simulink model "test_multi_bram_Delay"  (Simulink 7.6)
settings: Solver=ode45  StartTime=0.0  StopTime=10.0  RelTol=1e-3
libraries: xbsIndex_r4 x32, monroe_library x2, xps_library x1
settings Model: Creator=monroe  LastModifiedBy=monroe

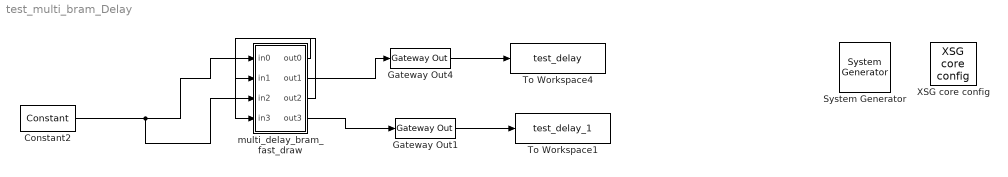
== system test_multi_bram_Delay ==
  " System Generator" : xbsIndex_r4/ System Generator  Tag=genX  SystemSampleTime=-1  xilinxfamily=virtex5  part=xc5vsx95t  speed=-1  package=ff1136  synthesis_tool=XST  clock_wrapper=Clock Enables  directory=./spec_2pol_4kw_6tap_pfb/sysgen  testbench=off  simulink_period=1  sysclk_period=2.6667  dcm_input_clock_period=100  incr_netlist=off  trim_vbits=Everywhere in SubSystem  dbl_ovrd=According to Block Masks  core_generation=According to Block Masks  run_coregen=off  deprecated_control=off  eval_field=0  block_type=sysgen
      settings: block_version=11.4
  Constant2 : xbsIndex_r4/Constant  arith_type=Signed (2's comp)  const=0.9  n_bits=8  bin_pt=7  explicit_period=on  period=1  equ=P=C  opselect=C  inp2=PCIN>>17  opr=+  inp1=P  carry=CIN  dbl_ovrd=off  block_type=constant
  Gateway Out1 : xbsIndex_r4/Gateway Out  hdl_port=on  timing_constraint=None  locs_specified=off  LOCs={}  block_type=gatewayout
      settings: infoedit="Gateway out block.  Converts Xilinx fixed point inputs into ouputs of type Simulink integer, double, or fixed point.<br><br>Hardware notes:  In hardware these blocks become top level output ports or are discarded, depending on how they are configured."  block_version=12.3
  Gateway Out4 : xbsIndex_r4/Gateway Out  hdl_port=on  timing_constraint=None  locs_specified=off  LOCs={}  block_type=gatewayout
      settings: infoedit="Gateway out block.  Converts Xilinx fixed point inputs into ouputs of type Simulink integer, double, or fixed point.<br><br>Hardware notes:  In hardware these blocks become top level output ports or are discarded, depending on how they are configured."  block_version=12.3
  To Workspace1 : ToWorkspace  VariableName=test_delay_1  SampleTime=-1  SaveFormat=Structure
  To Workspace4 : ToWorkspace  VariableName=test_delay  SampleTime=-1  SaveFormat=Structure
  XSG core config : xps_library/XSG core config  Tag=xps:xsg  SystemSampleTime=-1  hw_sys=ROACH:sx95t  ibob_linux=off  clk_src=adc0_clk  iBOB_clk_src=sys_clk  BEE2_ctrl_clk_src=sys_clk  BEE2_usr_clk_src=sys_clk  ROACH_clk_src=adc0_clk  CORR_clk_src=sys_clk  gpio_clk_io_group=iBOB:sma  gpio_clk_bit_index=0  clk_rate=375  sample_period=1  synthesis_tool=XST  mpc_type=powerpc440_ext
  multi_delay_bram_fast_draw : Subsystem
  wires:
  multi_delay_bram_fast_draw/3(out2) -> multi_delay_bram_fast_draw/4(in3)
  multi_delay_bram_fast_draw/1(out0) -> multi_delay_bram_fast_draw/2(in1)
  Constant2/1 -> multi_delay_bram_fast_draw/1(in0), multi_delay_bram_fast_draw/3(in2)
  Gateway Out4/1 -> To Workspace4/1
  Gateway Out1/1 -> To Workspace1/1
  multi_delay_bram_fast_draw/2(out1) -> Gateway Out4/1
  multi_delay_bram_fast_draw/4(out3) -> Gateway Out1/1

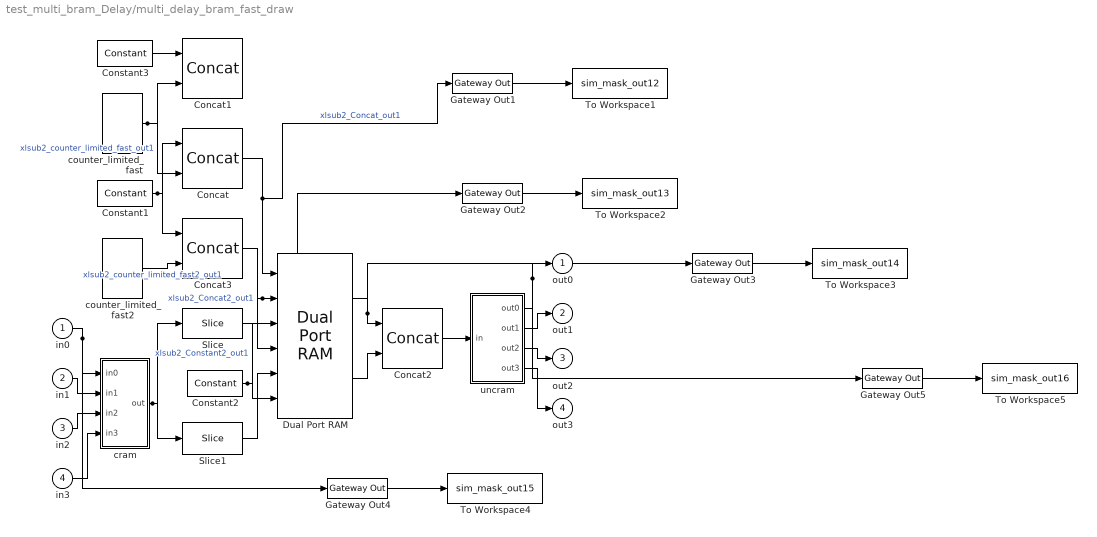
== system test_multi_bram_Delay/multi_delay_bram_fast_draw ==
  in0 : Inport
  in1 : Inport  Port=2
  in2 : Inport  Port=3
  in3 : Inport  Port=4
  Concat{,1..3} (4 alike) : xbsIndex_r4/Concat  num_inputs=2  dbl_ovrd=off  block_type=concat
  Constant1 : xbsIndex_r4/Constant  arith_type=Boolean  const=1  n_bits=1  bin_pt=0  explicit_period=on  period=1  equ=P=C  opselect=C  inp2=PCIN>>17  opr=+  inp1=P  carry=CIN  dbl_ovrd=off  block_type=constant
  Constant2 : xbsIndex_r4/Constant  arith_type=Boolean  const=1  n_bits=1  bin_pt=0  explicit_period=on  period=1  equ=P=C  opselect=C  inp2=PCIN>>17  opr=+  inp1=P  carry=CIN  dbl_ovrd=off  block_type=constant
  Constant3 : xbsIndex_r4/Constant  arith_type=Boolean  const=0  n_bits=1  bin_pt=0  explicit_period=on  period=1  equ=P=C  opselect=C  inp2=PCIN>>17  opr=+  inp1=P  carry=CIN  dbl_ovrd=off  block_type=constant
  Dual Port RAM : xbsIndex_r4/Dual Port RAM  depth=2048  initVector=0  distributed_mem=Block RAM  init_a=0  init_b=0  rst_a=off  rst_b=off  en_a=off  en_b=off  latency=2  write_mode_A=Read Before Write  write_mode_B=Read Before Write  dbl_ovrd=off  optimize=Area  use_rpm=on  block_type=dpram
  Gateway Out{1..5} (5 alike) : xbsIndex_r4/Gateway Out  hdl_port=on  timing_constraint=None  locs_specified=off  LOCs={}  block_type=gatewayout
      settings: infoedit="Gateway out block.  Converts Xilinx fixed point inputs into ouputs of type Simulink integer, double, or fixed point.<br><br>Hardware notes:  In hardware these blocks become top level output ports or are discarded, depending on how they are configured."  block_version=12.3
  Slice : xbsIndex_r4/Slice  nbits=16  boolean_output=off  mode=Upper Bit Location + Width  bit1=0  base1=MSB of Input  bit0=0  base0=MSB of Input  dbl_ovrd=off  block_type=slice
  Slice1 : xbsIndex_r4/Slice  nbits=16  boolean_output=off  mode=Upper Bit Location + Width  bit1=-16  base1=MSB of Input  bit0=0  base0=MSB of Input  dbl_ovrd=off  block_type=slice
  To Workspace1 : ToWorkspace  VariableName=sim_mask_out12  SampleTime=-1  SaveFormat=Structure
  To Workspace2 : ToWorkspace  VariableName=sim_mask_out13  SampleTime=-1  SaveFormat=Structure
  To Workspace3 : ToWorkspace  VariableName=sim_mask_out14  SampleTime=-1  SaveFormat=Structure
  To Workspace4 : ToWorkspace  VariableName=sim_mask_out15  SampleTime=-1  SaveFormat=Structure
  To Workspace5 : ToWorkspace  VariableName=sim_mask_out16  SampleTime=-1  SaveFormat=Structure
  counter_limited_fast : monroe_library/counter_limited_fast  SystemSampleTime=-1  bit_width=10  count_to=1021
  counter_limited_fast2 : monroe_library/counter_limited_fast  SystemSampleTime=-1  bit_width=10  count_to=1021
  cram : Subsystem
  uncram : Subsystem
  out0 : Outport
  out1 : Outport  Port=2
  out2 : Outport  Port=3
  out3 : Outport  Port=4
  wires:
  Gateway Out5/1 -> To Workspace5/1
  Gateway Out4/1 -> To Workspace4/1
  Gateway Out3/1 -> To Workspace3/1
  Gateway Out2/1 -> To Workspace2/1
  Gateway Out1/1 -> To Workspace1/1
  cram/1(out) -> Slice1/1, Slice/1
  counter_limited_fast/1 -> Concat1/2, Concat/2  "xlsub2_counter_limited_fast_out1"
  Constant1/1 -> Concat3/1, Concat/1
  Constant2/1 -> Dual Port RAM/6, Dual Port RAM/3  "xlsub2_Constant2_out1"
  uncram/4(out3) -> out3/1
  uncram/3(out2) -> out2/1
  uncram/2(out1) -> out1/1
  uncram/1(out0) -> Gateway Out5/1, out0/1
  Concat2/1 -> uncram/1(in)
  Dual Port RAM/2 -> Concat2/2
  Dual Port RAM/1 -> Gateway Out3/1, Concat2/1
  Slice1/1 -> Dual Port RAM/5
  Concat3/1 -> Dual Port RAM/4  "xlsub2_Concat2_out1"
  Slice/1 -> Gateway Out2/1, Dual Port RAM/2
  Concat/1 -> Gateway Out1/1, Dual Port RAM/1  "xlsub2_Concat_out1"
  Constant3/1 -> Concat1/1
  counter_limited_fast2/1 -> Concat3/2  "xlsub2_counter_limited_fast2_out1"
  in3/1 -> cram/4(in3)
  in2/1 -> cram/3(in2)
  in1/1 -> cram/2(in1)
  in0/1 -> Gateway Out4/1, cram/1(in0)

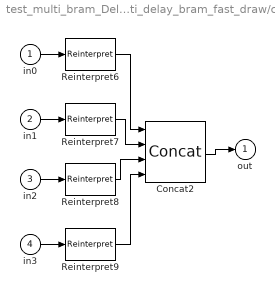
== system test_multi_bram_Delay/multi_delay_bram_fast_draw/cram ==
  in0 : Inport
  in1 : Inport  Port=2
  in2 : Inport  Port=3
  in3 : Inport  Port=4
  Concat2 : xbsIndex_r4/Concat  num_inputs=4  dbl_ovrd=off  block_type=concat
  Reinterpret{6..9} (4 alike) : xbsIndex_r4/Reinterpret  force_arith_type=on  arith_type=Unsigned  force_bin_pt=on  bin_pt=0  block_type=reinterpret
      settings: infoedit="Changes signal type without altering the binary representation.   You can changed the signal between signed and unsigned, and relocate the binary point.<br><br>Hardware notes: In hardware this block costs nothing.<br><br>Example:  Suppose the input is 6 bits wide, signed, with 2 fractional bits, and the output is forced to unsigned with 0 fractional bits.  Then an input of -2.0 (1110.00 in binary 2's complement) becomes an output of 56 (111000 in binary)."
  out : Outport
  wires:
  Reinterpret9/1 -> Concat2/4
  in3/1 -> Reinterpret9/1
  Reinterpret8/1 -> Concat2/3
  in2/1 -> Reinterpret8/1
  Reinterpret7/1 -> Concat2/2
  in1/1 -> Reinterpret7/1
  Reinterpret6/1 -> Concat2/1
  in0/1 -> Reinterpret6/1
  Concat2/1 -> out/1

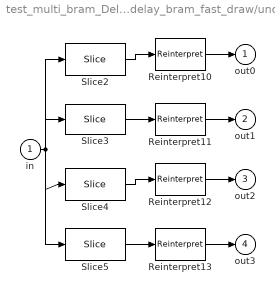
== system test_multi_bram_Delay/multi_delay_bram_fast_draw/uncram ==
  in : Inport
  Reinterpret{10..13} (4 alike) : xbsIndex_r4/Reinterpret  force_arith_type=on  arith_type="Signed  (2's comp)"  force_bin_pt=on  bin_pt=7  block_type=reinterpret
      settings: infoedit="Changes signal type without altering the binary representation.   You can changed the signal between signed and unsigned, and relocate the binary point.<br><br>Hardware notes: In hardware this block costs nothing.<br><br>Example:  Suppose the input is 6 bits wide, signed, with 2 fractional bits, and the output is forced to unsigned with 0 fractional bits.  Then an input of -2.0 (1110.00 in binary 2's complement) becomes an output of 56 (111000 in binary)."
  Slice2 : xbsIndex_r4/Slice  nbits=8  boolean_output=off  mode=Upper Bit Location + Width  bit1=-0  base1=MSB of Input  bit0=0  base0=MSB of Input  dbl_ovrd=off  block_type=slice
  Slice3 : xbsIndex_r4/Slice  nbits=8  boolean_output=off  mode=Upper Bit Location + Width  bit1=-8  base1=MSB of Input  bit0=0  base0=MSB of Input  dbl_ovrd=off  block_type=slice
  Slice4 : xbsIndex_r4/Slice  nbits=8  boolean_output=off  mode=Upper Bit Location + Width  bit1=-16  base1=MSB of Input  bit0=0  base0=MSB of Input  dbl_ovrd=off  block_type=slice
  Slice5 : xbsIndex_r4/Slice  nbits=8  boolean_output=off  mode=Upper Bit Location + Width  bit1=-24  base1=MSB of Input  bit0=0  base0=MSB of Input  dbl_ovrd=off  block_type=slice
  out0 : Outport
  out1 : Outport  Port=2
  out2 : Outport  Port=3
  out3 : Outport  Port=4
  wires:
  in/1 -> Slice5/1, Slice4/1, Slice3/1, Slice2/1
  Reinterpret13/1 -> out3/1
  Slice5/1 -> Reinterpret13/1
  Reinterpret12/1 -> out2/1
  Slice4/1 -> Reinterpret12/1
  Reinterpret11/1 -> out1/1
  Slice3/1 -> Reinterpret11/1
  Reinterpret10/1 -> out0/1
  Slice2/1 -> Reinterpret10/1
